simulink model "ACE9"  (R2021b)
settings: Solver=VariableStepAuto  StartTime=0.0  StopTime=10.0  RelTol=1e-3
settings Model: Creator=ACH  LastModifiedBy=ACH

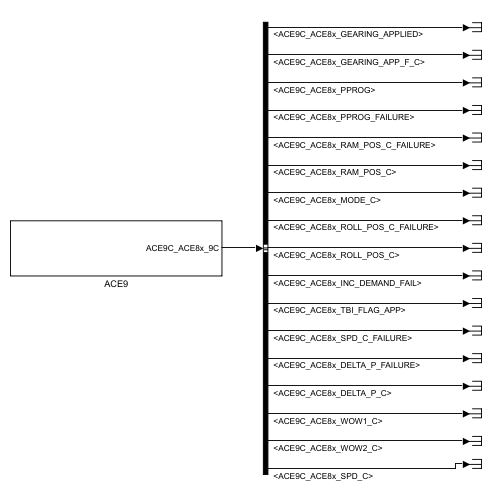
[thumbnail: Simulink's stored preview of the top-level diagram]
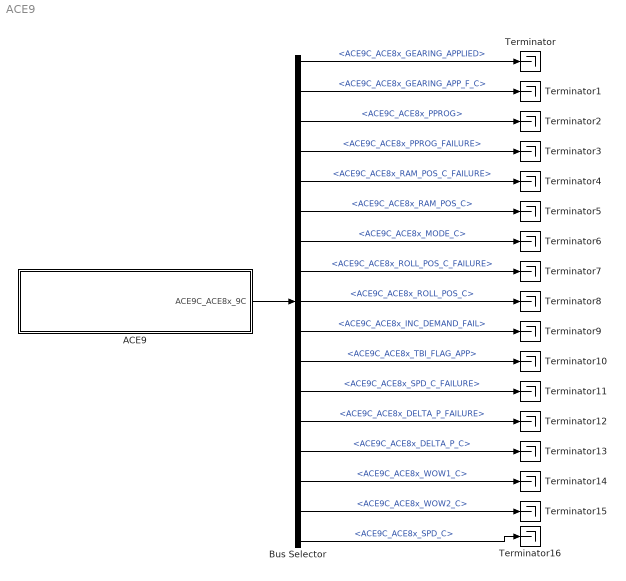
== system ACE9 ==
  ACE9 : Subsystem
  Bus Selector : BusSelector  OutputSignals=ACE9C_ACE8x_GEARING_APPLIED,ACE9C_ACE8x_GEARING_APP_F_C,ACE9C_ACE8x_PPROG,ACE9C_ACE8x_PPROG_FAILURE,ACE9C_ACE8x_RAM_POS_C_FAILURE,ACE9C_ACE8x_RAM_POS_C,ACE9C_ACE8x_MODE_C,ACE9C_ACE8x_ROLL_POS_C_FAILURE,ACE9C_ACE8x_ROLL_POS_C,ACE9C_ACE8x_INC_DEMAND_FAIL,ACE9C_ACE8x_TBI_FLAG_APP,ACE9C_ACE8x_SPD_C_FAILURE,ACE9C_ACE8x_DELTA_P_FAILURE,ACE9C_ACE8x_DELTA_P_C,ACE9C_ACE8x_WOW1_C,ACE9C_ACE8x_WOW2_C,ACE9C_ACE8x_SPD_C
  Terminator{,1..16} (17 alike) : Terminator
  wires:
  ACE9/1(ACE9C_ACE8x_9C) -> Bus Selector/1
  Bus Selector/1 -> Terminator/1  "<ACE9C_ACE8x_GEARING_APPLIED>"
  Bus Selector/2 -> Terminator1/1  "<ACE9C_ACE8x_GEARING_APP_F_C>"
  Bus Selector/3 -> Terminator2/1  "<ACE9C_ACE8x_PPROG>"
  Bus Selector/4 -> Terminator3/1  "<ACE9C_ACE8x_PPROG_FAILURE>"
  Bus Selector/5 -> Terminator4/1  "<ACE9C_ACE8x_RAM_POS_C_FAILURE>"
  Bus Selector/6 -> Terminator5/1  "<ACE9C_ACE8x_RAM_POS_C>"
  Bus Selector/7 -> Terminator6/1  "<ACE9C_ACE8x_MODE_C>"
  Bus Selector/8 -> Terminator7/1  "<ACE9C_ACE8x_ROLL_POS_C_FAILURE>"
  Bus Selector/9 -> Terminator8/1  "<ACE9C_ACE8x_ROLL_POS_C>"
  Bus Selector/10 -> Terminator9/1  "<ACE9C_ACE8x_INC_DEMAND_FAIL>"
  Bus Selector/11 -> Terminator10/1  "<ACE9C_ACE8x_TBI_FLAG_APP>"
  Bus Selector/12 -> Terminator11/1  "<ACE9C_ACE8x_SPD_C_FAILURE>"
  Bus Selector/13 -> Terminator12/1  "<ACE9C_ACE8x_DELTA_P_FAILURE>"
  Bus Selector/14 -> Terminator13/1  "<ACE9C_ACE8x_DELTA_P_C>"
  Bus Selector/15 -> Terminator14/1  "<ACE9C_ACE8x_WOW1_C>"
  Bus Selector/16 -> Terminator15/1  "<ACE9C_ACE8x_WOW2_C>"
  Bus Selector/17 -> Terminator16/1  "<ACE9C_ACE8x_SPD_C>"

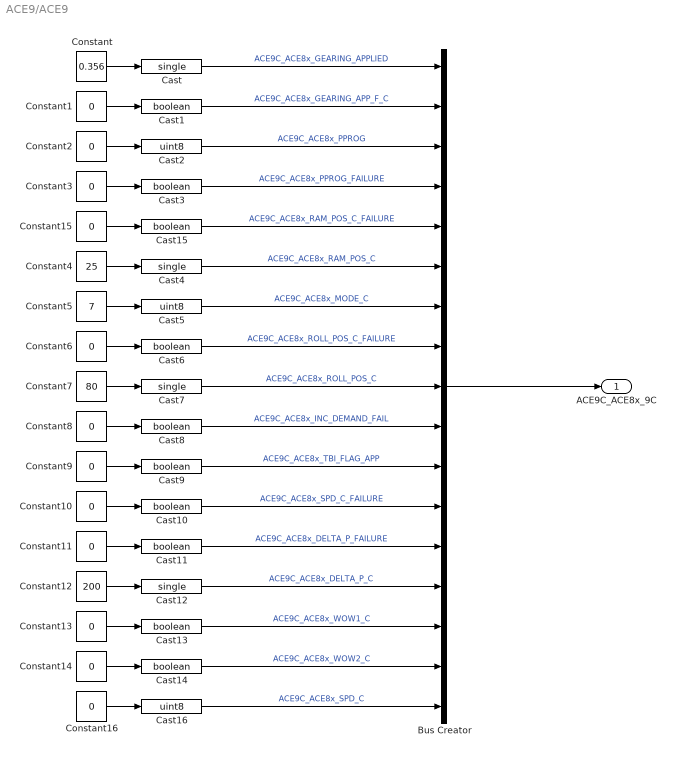
== system ACE9/ACE9 ==
  Bus Creator : BusCreator  Inputs=17  OutDataTypeStr=Bus: ACE9C_ACE8x_9C
      settings: InheritFromInputs=off
  Cast{,4,7,12} (4 alike) : DataTypeConversion  OutDataTypeStr=single
  Cast{1,3,6,8..11,13..15} (10 alike) : DataTypeConversion  OutDataTypeStr=boolean
  Cast16 : DataTypeConversion  OutDataTypeStr=uint8
  Cast2 : DataTypeConversion  OutDataTypeStr=uint8
  Cast5 : DataTypeConversion  OutDataTypeStr=uint8
  Constant : Constant  Value=0.356
  Constant{1..3,6,8..11,13..16} (12 alike) : Constant  Value=0
  Constant12 : Constant  Value=200
  Constant4 : Constant  Value=25
  Constant5 : Constant  Value=7
  Constant7 : Constant  Value=80
  ACE9C_ACE8x_9C : Outport
  wires:
  Constant4/1 -> Cast4/1
  Cast2/1 -> Bus Creator/3  "ACE9C_ACE8x_PPROG"
  Constant/1 -> Cast/1
  Constant16/1 -> Cast16/1
  Cast15/1 -> Bus Creator/5  "ACE9C_ACE8x_RAM_POS_C_FAILURE"
  Cast12/1 -> Bus Creator/14  "ACE9C_ACE8x_DELTA_P_C"
  Constant10/1 -> Cast10/1
  Constant9/1 -> Cast9/1
  Constant14/1 -> Cast14/1
  Constant7/1 -> Cast7/1
  Cast4/1 -> Bus Creator/6  "ACE9C_ACE8x_RAM_POS_C"
  Constant2/1 -> Cast2/1
  Constant12/1 -> Cast12/1
  Cast16/1 -> Bus Creator/17  "ACE9C_ACE8x_SPD_C"
  Constant6/1 -> Cast6/1
  Cast9/1 -> Bus Creator/11  "ACE9C_ACE8x_TBI_FLAG_APP"
  Cast14/1 -> Bus Creator/16  "ACE9C_ACE8x_WOW2_C"
  Constant5/1 -> Cast5/1
  Constant11/1 -> Cast11/1
  Cast1/1 -> Bus Creator/2  "ACE9C_ACE8x_GEARING_APP_F_C"
  Cast5/1 -> Bus Creator/7  "ACE9C_ACE8x_MODE_C"
  Cast6/1 -> Bus Creator/8  "ACE9C_ACE8x_ROLL_POS_C_FAILURE"
  Cast10/1 -> Bus Creator/12  "ACE9C_ACE8x_SPD_C_FAILURE"
  Cast7/1 -> Bus Creator/9  "ACE9C_ACE8x_ROLL_POS_C"
  Constant8/1 -> Cast8/1
  Cast8/1 -> Bus Creator/10  "ACE9C_ACE8x_INC_DEMAND_FAIL"
  Constant13/1 -> Cast13/1
  Cast13/1 -> Bus Creator/15  "ACE9C_ACE8x_WOW1_C"
  Cast11/1 -> Bus Creator/13  "ACE9C_ACE8x_DELTA_P_FAILURE"
  Constant3/1 -> Cast3/1
  Cast/1 -> Bus Creator/1  "ACE9C_ACE8x_GEARING_APPLIED"
  Cast3/1 -> Bus Creator/4  "ACE9C_ACE8x_PPROG_FAILURE"
  Constant15/1 -> Cast15/1
  Constant1/1 -> Cast1/1
  Bus Creator/1 -> ACE9C_ACE8x_9C/1
